simulink model "inject"  (Simulink 6.4)
settings: Solver=ode45  StartTime=0.0  StopTime=inf  RelTol=1e-3
settings Model: LastModifiedBy=Meg

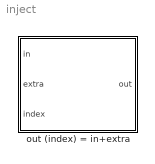
== system inject ==
  out (index) = in+extra : Stateflow chart

== matlab function out (index) = in+extra ==
  data: in input inherited; out output inherited; extra input inherited; index input inherited
function out = inject(in,extra,index)
% adds an EXTRA signal to specified elements (INDEX) of the IN vector

out = in;
for i=index
    out(i)=in(i)+extra;
end
